simulink model "SystemSpeedClosed"  (R2016b)
settings: Solver=ode45  StartTime=0.0  StopTime=1  RelTol=1e-3  EnableMultiTasking=on
libraries: powerlib x4, simulink x3, powerlib_meascontrol x1
settings Model: Creator=Administrator  LastModifiedBy=Administrator
settings DataIOCC: LimitDataPoints=on  SaveFormat=Array
settings OptimizationCC: LifeSpan=inf
settings DebuggingCC: SolverPrmCheckMsg=warning  InitInArrayFormatMsg=none  SFUnexpectedBacktrackingDiag=warning  SFNoUnconditionalDefaultTransitionDiag=warning  SFExecutionAtInitializationDiag=none
settings HardwareCC: ProdBitPerPointer=32  ProdBitPerSizeT=32  ProdBitPerPtrDiffT=32  ProdLargestAtomicFloat=None  ProdIntDivRoundTo=Undefined  ProdEndianess=Unspecified  ProdWordSize=32  ProdHWDeviceType=32-bit Generic
settings ModelReferenceCC: PropagateSignalLabelsOutOfModel=off
settings GRTTargetCC: TargetLangStandard=C89/C90 (ANSI)  GeneratePreprocessorConditionals=Disable all
settings ConfigComp: CovMetricSettings=dw  CovHtmlReporting=on  CovSaveCumulativeToWorkspaceVar=on  CovSaveSingleToWorkspaceVar=on  CovExternalEMLEnable=off  CovSFcnEnable=off

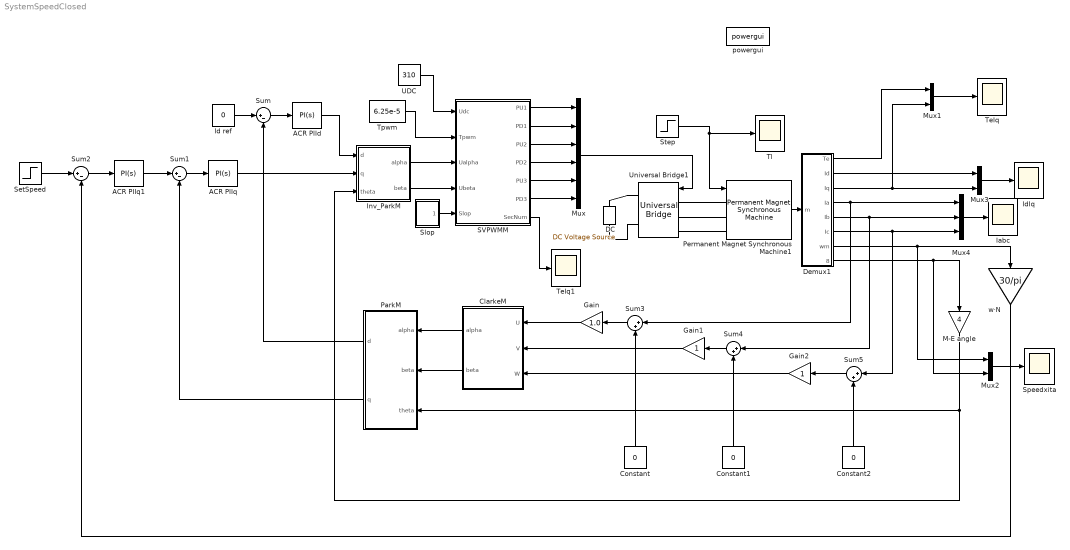
== system SystemSpeedClosed ==
  ACR PIId : simulink/Continuous/PID Controller  Controller=PI  TimeDomain=Continuous-time  SampleTime=-1  IntegratorMethod=Forward Euler  FilterMethod=Forward Euler  Form=Parallel  UseFilter=on  ControllerParametersSource=internal  P=45  I=23  D=0  N=100  InitialConditionSource=internal  InitialConditionForIntegrator=0  InitialConditionForFilter=0  ExternalReset=none  LimitOutput=off  UpperSaturationLimit=inf  LowerSaturationLimit=-inf  LinearizeAsGain=on  AntiWindupMode=none  Kb=1  TrackingMode=off  Kt=1  PParamMin=[]  PParamMax=[]  IParamMin=[]  IParamMax=[]  DParamMin=[]  DParamMax=[]  NParamMin=[]  NParamMax=[]  KbParamMin=[]  KbParamMax=[]  KtParamMin=[]  KtParamMax=[]  POutMin=[]  POutMax=[]  IOutMin=[]  IOutMax=[]  DOutMin=[]  DOutMax=[]  NOutMin=[]  NOutMax=[]  KbOutMin=[]  KbOutMax=[]  KtOutMin=[]  KtOutMax=[]  IntegratorOutMin=[]  IntegratorOutMax=[]  FilterOutMin=[]  FilterOutMax=[]  SumOutMin=[]  SumOutMax=[]  SumI1OutMin=[]  SumI1OutMax=[]  SumI2OutMin=[]  SumI2OutMax=[]  SumI3OutMin=[]  SumI3OutMax=[]  SumDOutMin=[]  SumDOutMax=[]  SaturationOutMin=[]  SaturationOutMax=[]  IntegratorContinuousStateAttributes=''  IntegratorStateMustResolveToSignalObject=off  IntegratorRTWStateStorageClass=Auto  FilterContinuousStateAttributes=''  FilterStateMustResolveToSignalObject=off  FilterRTWStateStorageClass=Auto  DifferentiatorICPrevScaledInput=0  DifferentiatorOutMin=[]  DifferentiatorOutMax=[]
  ACR PIIq : simulink/Continuous/PID Controller  Controller=PI  TimeDomain=Continuous-time  SampleTime=-1  IntegratorMethod=Forward Euler  FilterMethod=Forward Euler  Form=Parallel  UseFilter=on  ControllerParametersSource=internal  P=50  I=0.5  D=0  N=100  InitialConditionSource=internal  InitialConditionForIntegrator=0  InitialConditionForFilter=0  ExternalReset=none  LimitOutput=off  UpperSaturationLimit=inf  LowerSaturationLimit=-inf  LinearizeAsGain=on  AntiWindupMode=none  Kb=1  TrackingMode=off  Kt=1  PParamMin=[]  PParamMax=[]  IParamMin=[]  IParamMax=[]  DParamMin=[]  DParamMax=[]  NParamMin=[]  NParamMax=[]  KbParamMin=[]  KbParamMax=[]  KtParamMin=[]  KtParamMax=[]  POutMin=[]  POutMax=[]  IOutMin=[]  IOutMax=[]  DOutMin=[]  DOutMax=[]  NOutMin=[]  NOutMax=[]  KbOutMin=[]  KbOutMax=[]  KtOutMin=[]  KtOutMax=[]  IntegratorOutMin=[]  IntegratorOutMax=[]  FilterOutMin=[]  FilterOutMax=[]  SumOutMin=[]  SumOutMax=[]  SumI1OutMin=[]  SumI1OutMax=[]  SumI2OutMin=[]  SumI2OutMax=[]  SumI3OutMin=[]  SumI3OutMax=[]  SumDOutMin=[]  SumDOutMax=[]  SaturationOutMin=[]  SaturationOutMax=[]  IntegratorContinuousStateAttributes=''  IntegratorStateMustResolveToSignalObject=off  IntegratorRTWStateStorageClass=Auto  FilterContinuousStateAttributes=''  FilterStateMustResolveToSignalObject=off  FilterRTWStateStorageClass=Auto  DifferentiatorICPrevScaledInput=0  DifferentiatorOutMin=[]  DifferentiatorOutMax=[]
  ACR PIIq1 : simulink/Continuous/PID Controller  Controller=PI  TimeDomain=Continuous-time  SampleTime=-1  IntegratorMethod=Forward Euler  FilterMethod=Forward Euler  Form=Parallel  UseFilter=on  ControllerParametersSource=internal  P=0.3  I=0.002  D=0  N=100  InitialConditionSource=internal  InitialConditionForIntegrator=0  InitialConditionForFilter=0  ExternalReset=none  LimitOutput=off  UpperSaturationLimit=inf  LowerSaturationLimit=-inf  LinearizeAsGain=on  AntiWindupMode=none  Kb=1  TrackingMode=off  Kt=1  PParamMin=[]  PParamMax=[]  IParamMin=[]  IParamMax=[]  DParamMin=[]  DParamMax=[]  NParamMin=[]  NParamMax=[]  KbParamMin=[]  KbParamMax=[]  KtParamMin=[]  KtParamMax=[]  POutMin=[]  POutMax=[]  IOutMin=[]  IOutMax=[]  DOutMin=[]  DOutMax=[]  NOutMin=[]  NOutMax=[]  KbOutMin=[]  KbOutMax=[]  KtOutMin=[]  KtOutMax=[]  IntegratorOutMin=[]  IntegratorOutMax=[]  FilterOutMin=[]  FilterOutMax=[]  SumOutMin=[]  SumOutMax=[]  SumI1OutMin=[]  SumI1OutMax=[]  SumI2OutMin=[]  SumI2OutMax=[]  SumI3OutMin=[]  SumI3OutMax=[]  SumDOutMin=[]  SumDOutMax=[]  SaturationOutMin=[]  SaturationOutMax=[]  IntegratorContinuousStateAttributes=''  IntegratorStateMustResolveToSignalObject=off  IntegratorRTWStateStorageClass=Auto  FilterContinuousStateAttributes=''  FilterStateMustResolveToSignalObject=off  FilterRTWStateStorageClass=Auto  DifferentiatorICPrevScaledInput=0  DifferentiatorOutMin=[]  DifferentiatorOutMax=[]
  ClarkeM : MATLAB Function  TreatAsAtomicUnit=on
  Constant : Constant  Value=0
  Constant1 : Constant  Value=0
  Constant2 : Constant  Value=0
  DC : powerlib/Electrical Sources/DC Voltage Source  Amplitude=310  Measurements=None
  Demux1 : Subsystem
  Gain : Gain  Gain=1.0
  Gain1 : Gain
  Gain2 : Gain
  Iabc : Scope
  Id ref : Constant  Value=0
  IdIq : Scope
  Inv_ParkM : MATLAB Function  TreatAsAtomicUnit=on
  M-E angle : Gain  Gain=4
  Mux : Mux  Inputs=6
  Mux1 : Mux  Inputs=2
  Mux2 : Mux  Inputs=2
  Mux3 : Mux  Inputs=2
  Mux4 : Mux  Inputs=3
  ParkM : MATLAB Function  TreatAsAtomicUnit=on
  Permanent Magnet Synchronous Machine1 : powerlib/Machines/Permanent Magnet Synchronous Machine  NbPhases=3  FluxDistribution=Sinusoidal  RotorType=Round  MechanicalLoad=Torque Tm  PresetModel=No  ShowDetailedParameters=on  MeasurementBus=off  Resistance=1  Inductance=8.5e-3  dqInductances=[8.5e-3,8.5e-3]  La=0.01  MachineConstant=Flux linkage established by magnets (V.s)  Flux=0.1827  VoltageCst=132.5525  TorqueCst=1.0962  Flat=120  Mechanical=[0.006 0.0003035 4 0]  PolePairs=4  InitialConditions=[0,0, 0,0]  InitialConditions5ph=[0 0 0 0 0 0]  TsPowergui=0  TsBlock=-1  RefAngle=Aligned with phase A axis (original Park)
  SVPWMM : MATLAB Function  TreatAsAtomicUnit=on
  SetSpeed : Step  Time=0  Before=600  After=600  SampleTime=0
  Slop : Subsystem
  Speedxita : Scope
  Step : Step  Time=1.5  Before=0.3  SampleTime=0
  Sum : Sum  Inputs=|+-
  Sum1 : Sum  Inputs=|+-
  Sum2 : Sum  Inputs=|+-
  Sum3 : Sum  Inputs=|++
  Sum4 : Sum  Inputs=|++
  Sum5 : Sum  Inputs=|++
  TeIq : Scope
  TeIq1 : Scope
  Tl : Scope
  Tpwm : Constant  Value=6.25e-5
  UDC : Constant  Value=310
  Universal Bridge1 : powerlib/Power Electronics/Universal Bridge  Arms=3  SnubberResistance=1e5  SnubberCapacitance=inf  Device=IGBT / Diodes  Ron=1e-3  Lon=0  ForwardVoltages="[  0  0  ]"  ForwardVoltage=0  GTOparameters=[ 10e-6 , 20e-6 ]  IGBTparameters=[ 1e-6 , 2e-6 ]  Measurements=None  Measurements_2=None  converterType=Rectifier
  powergui : powerlib/powergui  SimulationMode=Continuous  SolverType=Tustin  SampleTime=50e-6  frequency=60  SPID=off  DisableSnubberDevices=off  DisableRonSwitches=off  DisableVfSwitches=off  SwTol=0  DisplayEquations=off  Interpol=off  ExternalGateDelay=off  methode=off  Ts=0  FunctionMessages=off  echomessages=off  HookPort=off  EnableUseOfTLC=off  x0status=blocks  frequencyindice=0  Pbase=100e6  ErrMax=1e-4  Iterations=50  UnitsV=kV  UnitsW=MW  buscounter=0  RestoreLinks=warning  ResistiveCurrentMeasurement=off  Frange=[0:2:500]  Ylog=off  Xlog=on  ShowGrid=off  save=off  variable=ZData  structure=0  ZoomFFT=on  StartTime=0.0  cycles=1  DisplayStyle=1  fundamental=60  FreqAxis=off  MaxFrequency=1000  frequencyindicesteady=1  RmsSteady=1  display=off
  w·N : Gain  Gain=30/pi
  wires:
  Mux/1 -> Universal Bridge1/1
  Demux1/8(thetam) -> Mux2/2, M-E angle/1
  Permanent Magnet Synchronous Machine1/1 -> Demux1/1(m)
  M-E angle/1 -> Inv_ParkM/3(theta), ParkM/3(theta)
  w·N/1 -> Sum2/2
  Demux1/5(Ib) -> Sum4/1, Mux4/2
  Demux1/6(Ic) -> Sum5/1, Mux4/3
  Demux1/3(Iq) -> Mux1/2, Mux3/2
  Demux1/2(Id) -> Mux3/1
  Demux1/4(Ia) -> Sum3/1, Mux4/1
  SVPWMM/1(PU1) -> Mux/1
  SVPWMM/2(PD1) -> Mux/2
  SVPWMM/3(PU2) -> Mux/3
  SVPWMM/4(PD2) -> Mux/4
  SVPWMM/5(PU3) -> Mux/5
  SVPWMM/6(PD3) -> Mux/6
  Slop/1(Out1) -> SVPWMM/5(Slop)
  UDC/1 -> SVPWMM/1(Udc)
  Tpwm/1 -> SVPWMM/2(Tpwm)
  ACR PIIq/1 -> Inv_ParkM/2(q)
  Inv_ParkM/1(alpha) -> SVPWMM/3(Ualpha)
  Inv_ParkM/2(beta) -> SVPWMM/4(Ubeta)
  Id ref/1 -> Sum/1
  ClarkeM/1(alpha) -> ParkM/1(alpha)
  ClarkeM/2(beta) -> ParkM/2(beta)
  ParkM/1(d) -> Sum/2
  Sum/1 -> ACR PIId/1
  ACR PIId/1 -> Inv_ParkM/1(d)
  Sum1/1 -> ACR PIIq/1
  ParkM/2(q) -> Sum1/2
  ACR PIIq1/1 -> Sum1/1
  SetSpeed/1 -> Sum2/1
  Mux1/1 -> TeIq/1
  Demux1/1(Te) -> Mux1/1
  Mux3/1 -> IdIq/1
  Demux1/7(wm) -> Mux2/1, w·N/1
  Mux2/1 -> Speedxita/1
  Sum2/1 -> ACR PIIq1/1
  Step/1 -> Tl/1, Permanent Magnet Synchronous Machine1/1
  Mux4/1 -> Iabc/1
  SVPWMM/7(SecNum) -> TeIq1/1
  Gain/1 -> ClarkeM/1(U)
  Gain1/1 -> ClarkeM/2(V)
  Gain2/1 -> ClarkeM/3(W)
  Sum3/1 -> Gain/1
  Sum4/1 -> Gain1/1
  Sum5/1 -> Gain2/1
  Constant/1 -> Sum3/2
  Constant1/1 -> Sum4/2
  Constant2/1 -> Sum5/2
  connections:
  Universal Bridge1/LConn1 -- Permanent Magnet Synchronous Machine1/LConn1
  Universal Bridge1/LConn2 -- Permanent Magnet Synchronous Machine1/LConn2
  Universal Bridge1/LConn3 -- Permanent Magnet Synchronous Machine1/LConn3
  Universal Bridge1/RConn2 -- DC/LConn1
  Universal Bridge1/RConn1 -- DC/RConn1

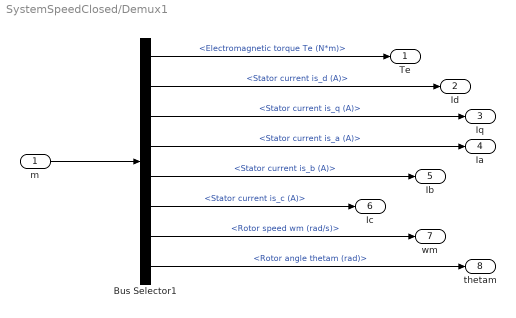
== system SystemSpeedClosed/Demux1 ==
  m : Inport
  Bus Selector1 : BusSelector  OutputSignals=Electromagnetic torque Te (N*m),Stator current is_d (A),Stator current is_q (A),Stator current is_a (A),Stator current is_b (A),Stator current is_c (A),Rotor speed wm (rad/s),Rotor angle thetam (rad)
  Te : Outport
  Id : Outport  Port=2
  Iq : Outport  Port=3
  Ia : Outport  Port=4
  Ib : Outport  Port=5
  Ic : Outport  Port=6
  wm : Outport  Port=7
  thetam : Outport  Port=8
  wires:
  m/1 -> Bus Selector1/1
  Bus Selector1/4 -> Ia/1  "<Stator current is_a (A)>"
  Bus Selector1/5 -> Ib/1  "<Stator current is_b (A)>"
  Bus Selector1/6 -> Ic/1  "<Stator current is_c (A)>"
  Bus Selector1/7 -> wm/1  "<Rotor speed wm (rad/s)>"
  Bus Selector1/8 -> thetam/1  "<Rotor angle thetam (rad)>"
  Bus Selector1/1 -> Te/1  "<Electromagnetic torque Te (N*m)>"
  Bus Selector1/2 -> Id/1  "<Stator current is_d (A)>"
  Bus Selector1/3 -> Iq/1  "<Stator current is_q (A)>"

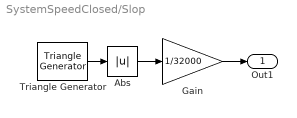
== system SystemSpeedClosed/Slop ==
  Abs : Abs
  Gain : Gain  Gain=1/32000
  Triangle Generator : powerlib_meascontrol/Pulse & Signal Generators/Triangle Generator  Freq=8e3  Phase=90  Ts=0
  Out1 : Outport
  wires:
  Triangle Generator/1 -> Abs/1
  Abs/1 -> Gain/1
  Gain/1 -> Out1/1

== matlab function SystemSpeedClosed/SVPWMM ==
  data: Udc input; Tpwm input; Ualpha input; PU1 output; PD1 output; PU2 output; PD2 output; PU3 output; PD3 output; Ubeta input; Slop input; SecNum output
function [PU1, PD1, PU2, PD2, PU3, PD3, SecNum] = SVPWM(Udc, Tpwm, Ualpha, Ubeta, Slop)
% Sector Cal %
if (Ubeta >= 0)
    if(Ualpha >= 0)
        if(sqrt(3)*Ualpha >= Ubeta)
            SecNum = 1;
        else
            SecNum = 2;
        end
    else
        if(Ubeta < (-sqrt(3)*Ualpha))
            SecNum = 3;
        else
            SecNum = 2;
        end
    end
else
    if(Ualpha < 0)
        if((-sqrt(3)*Ualpha) > (-Ubeta))
            SecNum = 4;
        else
            SecNum = 5;
        end
    else
        if(sqrt(3)*Ualpha > (-Ubeta))
            SecNum = 6;
        else
            SecNum = 5;
        end
    end
end

% Time Cal %
t1 = 0;
t2 = 0;
t0 = 0;
X = sqrt(2)*Tpwm*Ubeta / Udc;
Y = sqrt(2)*Tpwm*(Ubeta + sqrt(3)*Ualpha) / (2*Udc);
Z = sqrt(2)*Tpwm*(Ubeta - sqrt(3)*Ualpha) / (2*Udc);
switch SecNum
    case 1
        t1 = -Z;
        t2 = X;
     case 2
        t1 = Z;
        t2 = Y;
    case 3
        t1 = X;
        t2 = -Y;
    case 4
        t1 = -X;
        t2 = Z;
    case 5
        t1 = -Y;
        t2 = -Z;
    case 6
        t1 = Y;
        t2 = -X;
    otherwise
end

% Saturated treatment %
if((t1+t2) >= Tpwm)	
  t1 = t1 * Tpwm / (t1+t2);
  t2 = t2 * Tpwm / (t1+t2);
else
end
t0 = Tpwm - t1 - t2;
Ta = t0/4;
Tb = Ta + (t1/2);
Tc = Tb + (t2/2);

% Register Congiguration %
PU1 = 0;
PD1 = 0;
PU2 = 0;
PD2 = 0;
PU3 = 0;
PD3 = 0;
switch SecNum
    case 1
        if(Slop>=Ta)
            PU1 = 1;
            PD1 = 0;
        else
            PU1 = 0;
            PD1 = 1;
        end
        if(Slop>=Tb)
            PU2 = 1;
            PD2 = 0;
        else
            PU2 = 0;
            PD2 = 1;
        end
        if(Slop>=Tc)
            PU3 = 1;
            PD3 = 0;
        else
            PU3 = 0;
            PD3 = 1;
        end        
    case 2
        if(Slop>=Tb)
            PU1 = 1;
            PD1 = 0;
        else
            PU1 = 0;
            PD1 = 1;
        end
        if(Slop>=Ta)
            PU2 = 1;
            PD2 = 0;
        else
            PU2 = 0;
            PD2 = 1;
        end
        if(Slop>=Tc)
            PU3 = 1;
            PD3 = 0;
        else
            PU3 = 0;
            PD3 = 1;
        end  
    case 3
        if(Slop>=Tc)
            PU1 = 1;
            PD1 = 0;
        else
            PU1 = 0;
            PD1 = 1;
        end
        if(Slop>=Ta)
            PU2 = 1;
            PD2 = 0;
        else
            PU2 = 0;
            PD2 = 1;
        end
        if(Slop>=Tb)
            PU3 = 1;
            PD3 = 0;
        else
            PU3 = 0;
            PD3 = 1;
        end  
    case 4
        if(Slop>=Tc)
            PU1 = 1;
            PD1 = 0;
        else
            PU1 = 0;
            PD1 = 1;
        end
        if(Slop>=Tb)
            PU2 = 1;
            PD2 = 0;
        else
            PU2 = 0;
            PD2 = 1;
        end
        if(Slop>=Ta)
            PU3 = 1;
            PD3 = 0;
        else
            PU3 = 0;
            PD3 = 1;
        end  
    case 5
        if(Slop>=Tb)
            PU1 = 1;
            PD1 = 0;
        else
            PU1 = 0;
            PD1 = 1;
        end
        if(Slop>=Tc)
            PU2 = 1;
            PD2 = 0;
        else
            PU2 = 0;
            PD2 = 1;
        end
        if(Slop>=Ta)
            PU3 = 1;
            PD3 = 0;
        else
            PU3 = 0;
            PD3 = 1;
        end  
    case 6
        if(Slop>=Ta)
            PU1 = 1;
            PD1 = 0;
        else
            PU1 = 0;
            PD1 = 1;
        end
        if(Slop>=Tc)
            PU2 = 1;
            PD2 = 0;
        else
            PU2 = 0;
            PD2 = 1;
        end
        if(Slop>=Tb)
            PU3 = 1;
            PD3 = 0;
        else
            PU3 = 0;
            PD3 = 1;
        end  
    otherwise
end
end

== matlab function SystemSpeedClosed/ClarkeM ==
  data: U input; alpha output; V input; beta output; W input
function [alpha, beta] = ClakerM3(U, V, W)
%#codegen
alpha = (2*U - V - W)/sqrt(6);
beta  = (V - W)/sqrt(2);

== matlab function SystemSpeedClosed/ParkM ==
  data: alpha input; beta input; theta input; d output; q output
function [d, q] = ParkM(alpha, beta, theta)
%#codegen
d =  alpha*cos(theta) + beta*sin(theta);
q = -alpha*sin(theta) + beta*cos(theta);

== matlab function SystemSpeedClosed/Inv_ParkM ==
  data: d input; q input; alpha output; beta output; theta input
function [alpha, beta] = ParkM(d, q, theta)
%#codegen
alpha = d*cos(theta) - q*sin(theta);
beta  = d*sin(theta) + q*cos(theta);
